simulink model "sns_simscape_EI_test"  (R2025b)
settings: Solver=ode23t  StartTime=0.0  StopTime=0.3  RelTol=1e-3
libraries: SNS_lib x5, fl_lib x2, nesl_utility x1
settings Model: Creator=Ben  LastModifiedBy=Ben

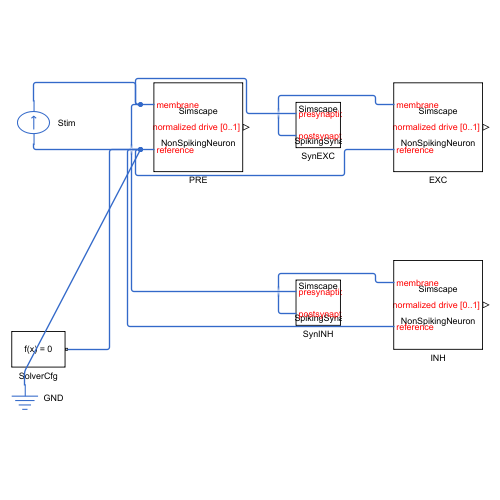
[thumbnail: Simulink's stored preview of the top-level diagram]
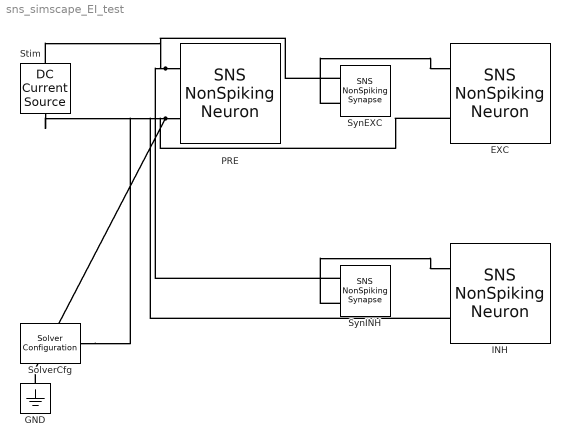
== system sns_simscape_EI_test ==
  EXC : SNS_lib/SNS NonSpiking Neuron  Vrest=-0.052 V  Gm=1e-7 S  Cm=5e-9 F  Thr=-0.045 V  Slope=1000 1/V
      settings: InternalSimscapePortConfiguration="{\"Bottom\":[],\"Left\":[{\"id\":\"m\",\"label\":\"membrane\",\"type\":\"foundation.electrical.electrical\"},{\"id\":\"r\",\"label\":\"reference\",\"type\":\"foundation.electrical.electrical\"}],\"Right\":[{\"id\":\"S\",\"label\":\"normalized drive [0..1]\",\"type\":\"output\"}],\"Top\":[]}"
  GND : fl_lib/Electrical/Electrical Elements/Electrical Reference
  INH : SNS_lib/SNS NonSpiking Neuron  Vrest=-0.052 V  Gm=1e-7 S  Cm=5e-9 F  Thr=-0.045 V  Slope=1000 1/V
      settings: InternalSimscapePortConfiguration="{\"Bottom\":[],\"Left\":[{\"id\":\"m\",\"label\":\"membrane\",\"type\":\"foundation.electrical.electrical\"},{\"id\":\"r\",\"label\":\"reference\",\"type\":\"foundation.electrical.electrical\"}],\"Right\":[{\"id\":\"S\",\"label\":\"normalized drive [0..1]\",\"type\":\"output\"}],\"Top\":[]}"
  PRE : SNS_lib/SNS NonSpiking Neuron  Vrest=-0.052 V  Gm=4e-7 S  Cm=5e-9 F  Thr=-0.045 V  Slope=1000 1/V
      settings: InternalSimscapePortConfiguration="{\"Bottom\":[],\"Left\":[{\"id\":\"m\",\"label\":\"membrane\",\"type\":\"foundation.electrical.electrical\"},{\"id\":\"r\",\"label\":\"reference\",\"type\":\"foundation.electrical.electrical\"}],\"Right\":[{\"id\":\"S\",\"label\":\"normalized drive [0..1]\",\"type\":\"output\"}],\"Top\":[]}"
  SolverCfg : nesl_utility/Solver Configuration  PhysicalDomain=network_engine_domain  SubClassName=solver  LeftPortType=input  RightPortType=generic  Tones=[]  Harmonics=[]  SimulateNoise=off  Profile=off  UseLocalSampling=off  EnableSwitchedLinearOptims=on  FrequencyDomain=off  UseCCode=off  RelTol=0.001  AbsTol=0.001  MinStep=1e-09  ToWorkspace=off  RevertToSquareIcSolve=off  NumHomotopyIterations=100  PhasorMode=off  PhasorModeNumHarmonics=1  ConsistencySolver=NEWTON_XTOL_AFTER_FTOL  IndexReductionMethod=DerivativeReplacement  DoDC=off  ResidualTolerance=1e-09  ConsistencyTolSource=GLOBAL  ConsistencyAbsTol=0.001  ConsistencyRelTol=0.001  ConsistencyTolFactor=0.001  UseLocalSolver=off  LocalSolverChoice=NE_BACKWARD_EULER_ADVANCER  ResolveIndetEquations=on  FunctionEvalNumThread=1  LocalSolverSampleTime=0.001  DoFixedCost=off  MaxNonlinIter=3  MaxModeIter=2  ComputeImpulses=off  ImpulseIterations=2  LinearAlgebra=auto  LinearAlgebraNumThread=0  EquationFormulation=NE_TIME_EF  DelaysMemoryBudget=1024  AutomaticFiltering=on  FilteringTimeConstant=0.001  PartitionStorageMethod=AS_NEEDED  PartitionMemoryBudget=1024  PartitionMethod=ROBUST  MultibodyUseLocalSolver=off  MultibodyLocalSolverChoice=ODE1  MultibodyLocalSolverSampleTime=0.001
  Stim : fl_lib/Electrical/Electrical Sources/DC Current Source  i0=4e-9 A
      settings: InternalSimscapePortConfiguration="{\"Bottom\":[],\"Left\":[{\"id\":\"p\",\"label\":\"\",\"type\":\"foundation.electrical.electrical\"}],\"Right\":[{\"id\":\"n\",\"label\":\"\",\"type\":\"foundation.electrical.electrical\"}],\"Top\":[]}"
  SynEXC : SNS_lib/SNS NonSpiking Synapse  gmax=1e-7 S  Esyn=0 V  ThrPre=-0.045 V  SlopePre=500 1/V  Isyn_specify=off  Isyn_priority=None  Isyn=0 A  Isyn_nominal_specify=off  Isyn_nominal_value=1  Isyn_nominal_unit=A  idst_specify=off  idst_priority=None  idst=0 A  idst_nominal_specify=off  idst_nominal_value=1  idst_nominal_unit=A
      settings: InternalSimscapePortConfiguration="{\"Bottom\":[],\"Left\":[{\"id\":\"p\",\"label\":\"presynaptic membrane node (sensed)\",\"type\":\"foundation.electrical.electrical\"},{\"id\":\"n\",\"label\":\"postsynaptic membrane node (driven)\",\"type\":\"foundation.electrical.electrical\"}],\"Right\":[],\"Top\":[]}"
  SynINH : SNS_lib/SNS NonSpiking Synapse  gmax=1e-7 S  Esyn=-0.072 V  ThrPre=-0.045 V  SlopePre=500 1/V  Isyn_specify=off  Isyn_priority=None  Isyn=0 A  Isyn_nominal_specify=off  Isyn_nominal_value=1  Isyn_nominal_unit=A  idst_specify=off  idst_priority=None  idst=0 A  idst_nominal_specify=off  idst_nominal_value=1  idst_nominal_unit=A
      settings: InternalSimscapePortConfiguration="{\"Bottom\":[],\"Left\":[{\"id\":\"p\",\"label\":\"presynaptic membrane node (sensed)\",\"type\":\"foundation.electrical.electrical\"},{\"id\":\"n\",\"label\":\"postsynaptic membrane node (driven)\",\"type\":\"foundation.electrical.electrical\"}],\"Right\":[],\"Top\":[]}"
  connections:
  Stim/LConn1 -- SynEXC/LConn1 -- PRE/LConn1 -- SynINH/LConn1
  Stim/RConn1 -- EXC/LConn2 -- INH/LConn2 -- GND/LConn1 -- PRE/LConn2 -- SolverCfg/RConn1
  SynEXC/LConn2 -- EXC/LConn1
  SynINH/LConn2 -- INH/LConn1
